simulink model "GuiHua"  (R2019a)
settings: Solver=VariableStepAuto  StartTime=0.0  StopTime=inf  RelTol=1e-3
undefined symbols (not defined in the file or in its folder): cal_P
libraries: simulink x2
settings Model: Creator=mi  LastModifiedBy=mi

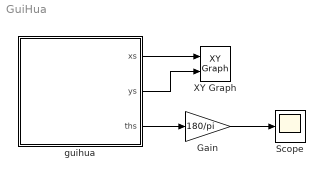
== system GuiHua ==
  Gain : Gain  Gain=180/pi
  Scope : Scope
  XY Graph : simulink/Sinks/XY Graph  xmin=-3  xmax=3  ymin=-0.2  ymax=5.2  st=-1
  "guihua " : Subsystem
  wires:
  "guihua "/1("xs ") -> XY Graph/1
  "guihua "/2("ys ") -> XY Graph/2
  "guihua "/3("ths ") -> Gain/1
  Gain/1 -> Scope/1

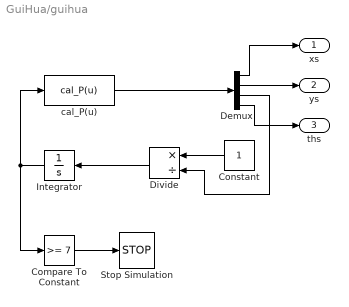
== system GuiHua/guihua  ==
  Compare To Constant : simulink/Logic and Bit Operations/Compare To Constant  relop=>=  const=7  OutDataTypeStr=boolean
  Constant : Constant
  Demux : Demux
  Divide : Product  Inputs=*/
  Integrator : Integrator
  Stop Simulation : Stop
  cal_P(u) : MATLABFcn  MATLABFcn=cal_P(u)  OutputDimensions=4
  "xs " : Outport
  "ys " : Outport  Port=2
  "ths " : Outport  Port=3
  wires:
  Constant/1 -> Divide/1
  Demux/3 -> Divide/2
  Integrator/1 -> Compare To Constant/1, cal_P(u)/1
  cal_P(u)/1 -> Demux/1
  Divide/1 -> Integrator/1
  Demux/2 -> "ys "/1
  Compare To Constant/1 -> Stop Simulation/1
  Demux/1 -> "xs "/1
  Demux/4 -> "ths "/1
